simulink model "heat_exchanger_disassembled"  (R2017b)
settings: Solver=VariableStepAuto  StartTime=0.0  StopTime=100  RelTol=1e-3
values from neighbouring files (symbols this model uses):
  Area = 20    [heat_exchanger_config.m]    (also in linearization.m)
  cp_H2O = 4190    [heat_exchanger_config.m]    (also in linearization.m)
  cp_wort = 4000    [heat_exchanger_config.m]    (also in linearization.m)
  HE_delay = 5    [heat_exchanger_config.m]    (also in linearization.m)
  m_H2O = 1    [heat_exchanger_config.m]    (also in linearization.m)
  m_wort = 1    [heat_exchanger_config.m]    (also in linearization.m)
  T_H2O_in = 10    [heat_exchanger_config.m]    (also in linearization.m)
  T_wort_in = 70    [heat_exchanger_config.m]    (also in linearization.m)
  U = 1000    [heat_exchanger_config.m]    (also in linearization.m)
libraries: simulink x2
settings Model: Creator=Alexander  LastModifiedBy=Alexander

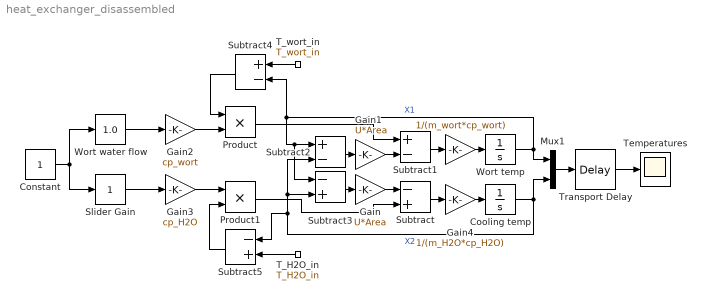
== system heat_exchanger_disassembled ==
  " " : Gain  Gain=1/(m_wort*cp_wort)
  Constant : Constant
  Cooling temp : Integrator  InitialCondition=T_H2O_in
  Gain : Gain  Gain=U*Area
  Gain1 : Gain  Gain=U*Area
  Gain2 : Gain  Gain=cp_wort
  Gain3 : Gain  Gain=cp_H2O
  Gain4 : Gain  Gain=1/(m_H2O*cp_H2O)
  Mux1 : Mux  Inputs=2
  Product : Product
  Product1 : Product
  Slider Gain : simulink/Math Operations/Slider Gain  gain=1  low=0  high=10
  Subtract : Sum  Inputs=-+
  Subtract1 : Sum  Inputs=+-
  Subtract2 : Sum  Inputs=+-
  Subtract3 : Sum  Inputs=-+
  Subtract4 : Sum  Inputs=+-
  Subtract5 : Sum  Inputs=-+
  T_H2O_in : Constant  Value=T_H2O_in
  T_wort_in : Constant  Value=T_wort_in
  Temperatures : Scope
  Transport Delay : TransportDelay  DelayTime=HE_delay
  Wort temp : Integrator  InitialCondition=T_wort_in
  Wort water flow : simulink/Math Operations/Slider Gain  gain=1.0  low=0  high=10
  wires:
  Transport Delay/1 -> Temperatures/1
  Cooling temp/1 -> Subtract5/1, Subtract3/2, Subtract2/2, Mux1/2  "X2"
  Wort temp/1 -> Subtract4/2, Subtract3/1, Subtract2/1, Mux1/1  "X1"
  Mux1/1 -> Transport Delay/1
  Gain1/1 -> Subtract1/2
  Gain/1 -> Subtract/1
  Subtract2/1 -> Gain1/1
  Subtract3/1 -> Gain/1
  Constant/1 -> Slider Gain/1, Wort water flow/1
  " "/1 -> Wort temp/1
  Subtract1/1 -> " "/1
  Gain4/1 -> Cooling temp/1
  Subtract/1 -> Gain4/1
  Wort water flow/1 -> Gain2/1
  T_wort_in/1 -> Subtract4/1
  Subtract4/1 -> Product/1
  Gain2/1 -> Product/2
  Product/1 -> Subtract1/1
  T_H2O_in/1 -> Subtract5/2
  Subtract5/1 -> Product1/2
  Gain3/1 -> Product1/1
  Product1/1 -> Subtract/2
  Slider Gain/1 -> Gain3/1
